simulink subsystem "TauDepolarLookup_Subsys"  (R2022b)
settings: Solver=VariableStepAuto  StartTime=0.0  StopTime=10.0  RelTol=1e-3
undefined symbols (not defined in the file): KaSoc_degC_tempLut, KaSoc_frc_socLut, KaSoc_sec_tauDepolarLut, SEC_TO_MILLISEC
settings Model: Creator=Niharika  LastModifiedBy=Niharika

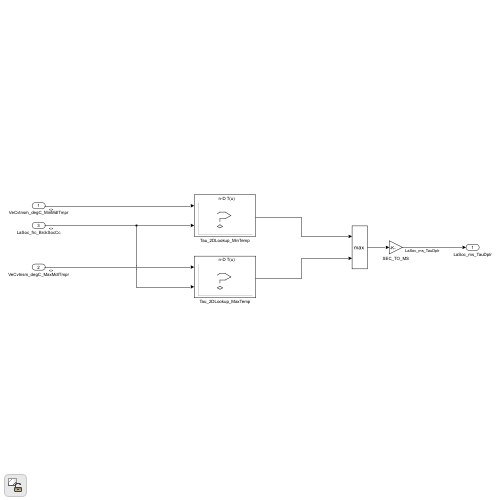
[thumbnail: Simulink's stored preview of the top-level diagram]
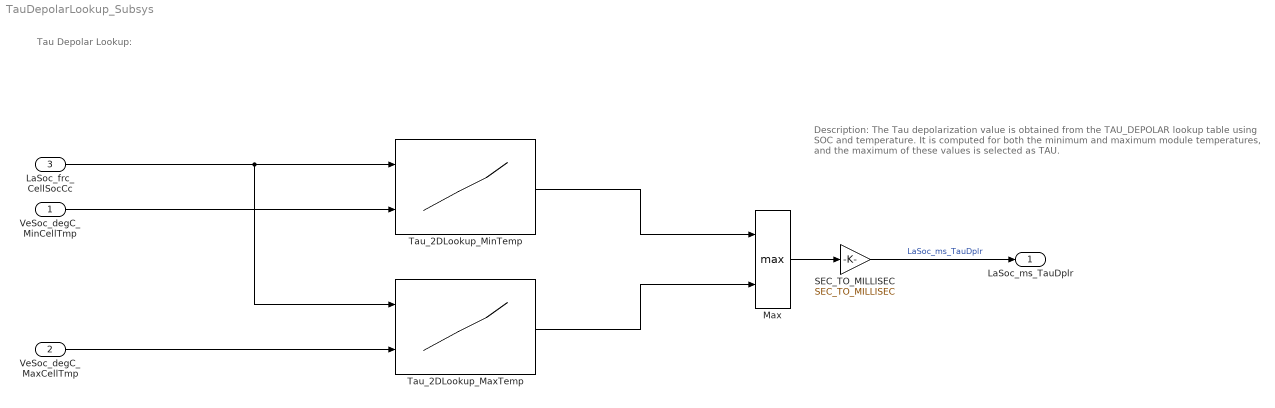
== system TauDepolarLookup_Subsys ==
  note: Tau Depolar Lookup:
  note: Description:
      | The Tau depolarization value is obtained from the TAU_DEPOLAR lookup table using SOC and temperature. It is computed for both the minimum and maximum module temperatures, and the maximum of these values is selected as TAU.
  VeSoc_degC_MinCellTmp : Inport
  VeSoc_degC_MaxCellTmp : Inport  Port=2
  LaSoc_frc_CellSocCc : Inport  Port=3
  Max : MinMax  Function=max  Inputs=2
  SEC_TO_MILLISEC : Gain  Gain=SEC_TO_MILLISEC
  Tau_2DLookup_MaxTemp : Lookup_n-D  BreakpointsForDimension1=KaSoc_frc_socLut  BreakpointsForDimension2=KaSoc_degC_tempLut  Table=KaSoc_sec_tauDepolarLut  ExtrapMethod=Clip  UseLastTableValue=on  InternalRulePriority=Speed  RndMeth=Simplest
      settings: InputPortMap=u0,u1
  Tau_2DLookup_MinTemp : Lookup_n-D  BreakpointsForDimension1=KaSoc_frc_socLut  BreakpointsForDimension2=KaSoc_degC_tempLut  Table=KaSoc_sec_tauDepolarLut  ExtrapMethod=Clip  UseLastTableValue=on  InternalRulePriority=Speed  RndMeth=Simplest
      settings: InputPortMap=u0,u1
  LaSoc_ms_TauDplr : Outport
  wires:
  Max/1 -> SEC_TO_MILLISEC/1
  SEC_TO_MILLISEC/1 -> LaSoc_ms_TauDplr/1  "LaSoc_ms_TauDplr"
  Tau_2DLookup_MinTemp/1 -> Max/1
  Tau_2DLookup_MaxTemp/1 -> Max/2
  VeSoc_degC_MaxCellTmp/1 -> Tau_2DLookup_MaxTemp/2
  LaSoc_frc_CellSocCc/1 -> Tau_2DLookup_MinTemp/1, Tau_2DLookup_MaxTemp/1
  VeSoc_degC_MinCellTmp/1 -> Tau_2DLookup_MinTemp/2
